simulink library "inp"  (R2021b)
settings: Solver=VariableStepAuto  StartTime=0.0  StopTime=10.0  RelTol=1e-3
undefined symbols (not defined in the file): C_TASK_5MS_S, FALSE, KINP_AcoreReadyToSlp_flg_ovrdflg, KINP_AcoreReadyToSlp_flg_ovrdval, KINP_AllowMovThd_OTA_enum_ovrdflg, KINP_AllowMovThd_OTA_enum_ovrdval, KINP_APSAngleTarget_Deg_ovrdflg, KINP_APSAngleTarget_Deg_ovrdval, KINP_APSDecReq_mps2_ovrdflg, KINP_APSDecReq_mps2_ovrdval, KINP_APSDecReqA_flg_ovrdflg, KINP_APSDecReqA_flg_ovrdval, KINP_APSDFLL_cm_ovrdflg, KINP_APSDFLL_cm_ovrdval, KINP_APSDFLR_cm_ovrdflg, KINP_APSDFLR_cm_ovrdval, KINP_APSDRLL_cm_ovrdflg, KINP_APSDRLL_cm_ovrdval, KINP_APSDRLR_cm_ovrdflg, KINP_APSDRLR_cm_ovrdval, KINP_APSExitCondition_enum_ovrdflg, KINP_APSExitCondition_enum_ovrdval, KINP_APSHWVer_enum_ovrdflg, KINP_APSHWVer_enum_ovrdval, KINP_APSProgressPCT_pct_ovrdflg, KINP_APSProgressPCT_pct_ovrdval, KINP_APSPwrReq_enum_ovrdflg, KINP_APSPwrReq_enum_ovrdval, KINP_APSReq_enum_ovrdflg, KINP_APSReq_enum_ovrdval, KINP_APSRQDisplay_enum_ovrdflg, KINP_APSRQDisplay_enum_ovrdval, KINP_APSRqEPASCtrl_flg_ovrdflg, KINP_APSRqEPASCtrl_flg_ovrdval, KINP_APSShiftPosnReq_enum_ovrdval, KINP_APSShiftPosnReq_enum_ovrflg, KINP_APSSpeedCMD_kph_ovrdval, KINP_APSSpeedCMD_kph_ovrflg, KINP_APSStaSystem_enum_ovrdflg, KINP_APSStaSystem_enum_ovrdval, KINP_APSSWVer_enum_ovrdflg, KINP_APSSWVer_enum_ovrdval, KINP_APSVMCReqA_flg_ovrdval, KINP_APSVMCReqA_flg_ovrflg, KINP_APSVRqEPASCtrl_flg_ovrdflg, KINP_APSVRqEPASCtrl_flg_ovrdval, KINP_AuxBattVolmV_mV_ovrdflg, KINP_AuxBattVolmV_mV_ovrdval, KINP_CAASSta_enum_ovrdflg, KINP_CAASSta_enum_ovrdval, KINP_CAASVMCReqA_flg_ovrdval, KINP_CAASVMCReqA_flg_ovrflg, KINP_CAN1BusOff_flg_ovrdflg, KINP_CAN1BusOff_flg_ovrdval, KINP_CAN2BusOff_flg_ovrdflg, KINP_CAN2BusOff_flg_ovrdval, KINP_CAN3BusOff_flg_ovrdflg, KINP_CAN3BusOff_flg_ovrdval, KINP_CAN4BusOff_flg_ovrdflg, KINP_CAN4BusOff_flg_ovrdval ... (+152)
libraries: FVT_lib x1035, hcu_lib x1
(part 28 of 33)

== system inp/INP/CAN4/SignalCheck/ZONE_FR_VCU ==
  BHAL_outputs : Inport
  inp_CanValid_bus : Inport  Port=2
  AGSErr : FVT_lib/inp/can_signal_template  SystemSampleTime=-1  VariantActivationTime=update diagram  Latency=0  AutoFrameSizeCalculation=off
      link override defval: Value=KINP_AGSErr_enum_defval
      link override ovrdflg: Value=KINP_AGSErr_enum_ovrdflg
      link override ovrdval: Value=KINP_AGSErr_enum_ovrdval
  BatInTemp : FVT_lib/inp/can_signal_template  SystemSampleTime=-1  VariantActivationTime=update diagram  Latency=0  AutoFrameSizeCalculation=off
      link override defval: Value=KINP_BatInTemp_C_defval
      link override ovrdflg: Value=KINP_BatInTemp_C_ovrdflg
      link override ovrdval: Value=KINP_BatInTemp_C_ovrdval
  BatInTempErr : FVT_lib/inp/can_signal_template  SystemSampleTime=-1  VariantActivationTime=update diagram  Latency=0  AutoFrameSizeCalculation=off
      link override defval: Value=KINP_BatInTempErr_enum_defval
      link override ovrdflg: Value=KINP_BatInTempErr_enum_ovrdflg
      link override ovrdval: Value=KINP_BatInTempErr_enum_ovrdval
  BatOutTemp : FVT_lib/inp/can_signal_template  SystemSampleTime=-1  VariantActivationTime=update diagram  Latency=0  AutoFrameSizeCalculation=off
      link override defval: Value=KINP_BatOutTemp_C_defval
      link override ovrdflg: Value=KINP_BatOutTemp_C_ovrdflg
      link override ovrdval: Value=KINP_BatOutTemp_C_ovrdval
  COMPErr : FVT_lib/inp/can_signal_template  SystemSampleTime=-1  VariantActivationTime=update diagram  Latency=0  AutoFrameSizeCalculation=off
      link override defval: Value=KINP_COMPErr_enum_defval
      link override ovrdflg: Value=KINP_COMPErr_enum_ovrdflg
      link override ovrdval: Value=KINP_COMPErr_enum_ovrdval
  EACProtectEnable : FVT_lib/inp/can_signal_template  SystemSampleTime=-1  VariantActivationTime=update diagram  Latency=0  AutoFrameSizeCalculation=off
      link override defval: Value=KINP_EACProtectEnable_enum_defval
      link override ovrdflg: Value=KINP_EACProtectEnable_enum_ovrdflg
      link override ovrdval: Value=KINP_EACProtectEnable_enum_ovrdval
  EWP3Err : FVT_lib/inp/can_signal_template  SystemSampleTime=-1  VariantActivationTime=update diagram  Latency=0  AutoFrameSizeCalculation=off
      link override defval: Value=KINP_EWP3Err_enum_defval
      link override ovrdflg: Value=KINP_EWP3Err_enum_ovrdflg
      link override ovrdval: Value=KINP_EWP3Err_enum_ovrdval
  EXV1Err : FVT_lib/inp/can_signal_template  SystemSampleTime=-1  VariantActivationTime=update diagram  Latency=0  AutoFrameSizeCalculation=off
      link override defval: Value=KINP_EXV1Err_enum_defval
      link override ovrdflg: Value=KINP_EXV1Err_enum_ovrdflg
      link override ovrdval: Value=KINP_EXV1Err_enum_ovrdval
  EXV2Err : FVT_lib/inp/can_signal_template  SystemSampleTime=-1  VariantActivationTime=update diagram  Latency=0  AutoFrameSizeCalculation=off
      link override defval: Value=KINP_EXV2Err_enum_defval
      link override ovrdflg: Value=KINP_EXV2Err_enum_ovrdflg
      link override ovrdval: Value=KINP_EXV2Err_enum_ovrdval
  FanErr : FVT_lib/inp/can_signal_template  SystemSampleTime=-1  VariantActivationTime=update diagram  Latency=0  AutoFrameSizeCalculation=off
      link override defval: Value=KINP_FanErr_enum_defval
      link override ovrdflg: Value=KINP_FanErr_enum_ovrdflg
      link override ovrdval: Value=KINP_FanErr_enum_ovrdval
  FrPMMLimpHomeActReq : FVT_lib/inp/can_signal_template  SystemSampleTime=-1  VariantActivationTime=update diagram  Latency=0  AutoFrameSizeCalculation=off
      link override defval: Value=KINP_FrPMMLimpHomeActReq_flg_defval
      link override ovrdflg: Value=KINP_FrPMMLimpHomeActReq_flg_ovrdflg
      link override ovrdval: Value=KINP_FrPMMLimpHomeActReq_flg_ovrdval
  MotorInTemp : FVT_lib/inp/can_signal_template  SystemSampleTime=-1  VariantActivationTime=update diagram  Latency=0  AutoFrameSizeCalculation=off
      link override defval: Value=KINP_MotorInTemp_C_defval
      link override ovrdflg: Value=KINP_MotorInTemp_C_ovrdflg
      link override ovrdval: Value=KINP_MotorInTemp_C_ovrdval
  MotorInTempErr : FVT_lib/inp/can_signal_template  SystemSampleTime=-1  VariantActivationTime=update diagram  Latency=0  AutoFrameSizeCalculation=off
      link override defval: Value=KINP_MotorInTempErr_enum_defval
      link override ovrdflg: Value=KINP_MotorInTempErr_enum_ovrdflg
      link override ovrdval: Value=KINP_MotorInTempErr_enum_ovrdval
  MotorOutTemp : FVT_lib/inp/can_signal_template  SystemSampleTime=-1  VariantActivationTime=update diagram  Latency=0  AutoFrameSizeCalculation=off
      link override defval: Value=KINP_MotorOutTemp_C_defval
      link override ovrdflg: Value=KINP_MotorOutTemp_C_ovrdflg
      link override ovrdval: Value=KINP_MotorOutTemp_C_ovrdval
  MotorOutTempErr : FVT_lib/inp/can_signal_template  SystemSampleTime=-1  VariantActivationTime=update diagram  Latency=0  AutoFrameSizeCalculation=off
      link override defval: Value=KINP_MotorOutTempErr_enum_defval
      link override ovrdflg: Value=KINP_MotorOutTempErr_enum_ovrdflg
      link override ovrdval: Value=KINP_MotorOutTempErr_enum_ovrdval
  PTHighP : FVT_lib/inp/can_signal_template  SystemSampleTime=-1  VariantActivationTime=update diagram  Latency=0  AutoFrameSizeCalculation=off
      link override defval: Value=KINP_PTHighP_KPa_defval
      link override ovrdflg: Value=KINP_PTHighP_KPa_ovrdflg
      link override ovrdval: Value=KINP_PTHighP_KPa_ovrdval
  PTHighPErr : FVT_lib/inp/can_signal_template  SystemSampleTime=-1  VariantActivationTime=update diagram  Latency=0  AutoFrameSizeCalculation=off
      link override defval: Value=KINP_PTHighPErr_enum_defval
      link override ovrdflg: Value=KINP_PTHighPErr_enum_ovrdflg
      link override ovrdval: Value=KINP_PTHighPErr_enum_ovrdval
  PTHighTact : FVT_lib/inp/can_signal_template  SystemSampleTime=-1  VariantActivationTime=update diagram  Latency=0  AutoFrameSizeCalculation=off
      link override defval: Value=KINP_PTHighTact_C_defval
      link override ovrdflg: Value=KINP_PTHighTact_C_ovrdflg
      link override ovrdval: Value=KINP_PTHighTact_C_ovrdval
  PTHighTactErr : FVT_lib/inp/can_signal_template  SystemSampleTime=-1  VariantActivationTime=update diagram  Latency=0  AutoFrameSizeCalculation=off
      link override defval: Value=KINP_PTHighTactErr_enum_defval
      link override ovrdflg: Value=KINP_PTHighTactErr_enum_ovrdflg
      link override ovrdval: Value=KINP_PTHighTactErr_enum_ovrdval
  PTLowP1 : FVT_lib/inp/can_signal_template  SystemSampleTime=-1  VariantActivationTime=update diagram  Latency=0  AutoFrameSizeCalculation=off
      link override defval: Value=KINP_PTLowP1_KPa_defval
      link override ovrdflg: Value=KINP_PTLowP1_KPa_ovrdflg
      link override ovrdval: Value=KINP_PTLowP1_KPa_ovrdval
  PTLowP1Err : FVT_lib/inp/can_signal_template  SystemSampleTime=-1  VariantActivationTime=update diagram  Latency=0  AutoFrameSizeCalculation=off
      link override defval: Value=KINP_PTLowP1Err_enum_defval
      link override ovrdflg: Value=KINP_PTLowP1Err_enum_ovrdflg
      link override ovrdval: Value=KINP_PTLowP1Err_enum_ovrdval
  PTLowP2 : FVT_lib/inp/can_signal_template  SystemSampleTime=-1  VariantActivationTime=update diagram  Latency=0  AutoFrameSizeCalculation=off
      link override defval: Value=KINP_PTLowP2_KPa_defval
      link override ovrdflg: Value=KINP_PTLowP2_KPa_ovrdflg
      link override ovrdval: Value=KINP_PTLowP2_KPa_ovrdval
  PTLowP2Err : FVT_lib/inp/can_signal_template  SystemSampleTime=-1  VariantActivationTime=update diagram  Latency=0  AutoFrameSizeCalculation=off
      link override defval: Value=KINP_PTLowP2Err_enum_defval
      link override ovrdflg: Value=KINP_PTLowP2Err_enum_ovrdflg
      link override ovrdval: Value=KINP_PTLowP2Err_enum_ovrdval
  PTLowT1 : FVT_lib/inp/can_signal_template  SystemSampleTime=-1  VariantActivationTime=update diagram  Latency=0  AutoFrameSizeCalculation=off
      link override defval: Value=KINP_PTLowT1_C_defval
      link override ovrdflg: Value=KINP_PTLowT1_C_ovrdflg
      link override ovrdval: Value=KINP_PTLowT1_C_ovrdval
  PTLowT1Err : FVT_lib/inp/can_signal_template  SystemSampleTime=-1  VariantActivationTime=update diagram  Latency=0  AutoFrameSizeCalculation=off
      link override defval: Value=KINP_PTLowT1Err_enum_defval
      link override ovrdflg: Value=KINP_PTLowT1Err_enum_ovrdflg
      link override ovrdval: Value=KINP_PTLowT1Err_enum_ovrdval
  PTLowT2 : FVT_lib/inp/can_signal_template  SystemSampleTime=-1  VariantActivationTime=update diagram  Latency=0  AutoFrameSizeCalculation=off
      link override defval: Value=KINP_PTLowT2_C_defval
      link override ovrdflg: Value=KINP_PTLowT2_C_ovrdflg
      link override ovrdval: Value=KINP_PTLowT2_C_ovrdval
  PTLowT2Err : FVT_lib/inp/can_signal_template  SystemSampleTime=-1  VariantActivationTime=update diagram  Latency=0  AutoFrameSizeCalculation=off
      link override defval: Value=KINP_PTLowT2Err_enum_defval
      link override ovrdflg: Value=KINP_PTLowT2Err_enum_ovrdflg
      link override ovrdval: Value=KINP_PTLowT2Err_enum_ovrdval
  SOTXVErr : FVT_lib/inp/can_signal_template  SystemSampleTime=-1  VariantActivationTime=update diagram  Latency=0  AutoFrameSizeCalculation=off
      link override defval: Value=KINP_SOTXVErr_enum_defval
      link override ovrdflg: Value=KINP_SOTXVErr_enum_ovrdflg
      link override ovrdval: Value=KINP_SOTXVErr_enum_ovrdval
  SOV1Err : FVT_lib/inp/can_signal_template  SystemSampleTime=-1  VariantActivationTime=update diagram  Latency=0  AutoFrameSizeCalculation=off
      link override defval: Value=KINP_SOV1Err_enum_defval
      link override ovrdflg: Value=KINP_SOV1Err_enum_ovrdflg
      link override ovrdval: Value=KINP_SOV1Err_enum_ovrdval
  SOV2Err : FVT_lib/inp/can_signal_template  SystemSampleTime=-1  VariantActivationTime=update diagram  Latency=0  AutoFrameSizeCalculation=off
      link override defval: Value=KINP_SOV2Err_enum_defval
      link override ovrdflg: Value=KINP_SOV2Err_enum_ovrdflg
      link override ovrdval: Value=KINP_SOV2Err_enum_ovrdval
  SOV3Err : FVT_lib/inp/can_signal_template  SystemSampleTime=-1  VariantActivationTime=update diagram  Latency=0  AutoFrameSizeCalculation=off
      link override defval: Value=KINP_SOV3Err_enum_defval
      link override ovrdflg: Value=KINP_SOV3Err_enum_ovrdflg
      link override ovrdval: Value=KINP_SOV3Err_enum_ovrdval
  Tamb : FVT_lib/inp/can_signal_template  SystemSampleTime=-1  VariantActivationTime=update diagram  Latency=0  AutoFrameSizeCalculation=off
      link override defval: Value=KINP_Tamb_C_defval
      link override ovrdflg: Value=KINP_Tamb_C_ovrdflg
      link override ovrdval: Value=KINP_Tamb_C_ovrdval
  TambErr : FVT_lib/inp/can_signal_template  SystemSampleTime=-1  VariantActivationTime=update diagram  Latency=0  AutoFrameSizeCalculation=off
      link override defval: Value=KINP_TambErr_enum_defval
      link override ovrdflg: Value=KINP_TambErr_enum_ovrdflg
      link override ovrdval: Value=KINP_TambErr_enum_ovrdval
  Terminator_{1..33} (33 alike) : Terminator
  True_VHAL_AGSErr_enum : Constant  Value=TRUE  OutDataTypeStr=boolean
  True_VHAL_BatInTempErr_enum : Constant  Value=TRUE  OutDataTypeStr=boolean
  True_VHAL_BatInTemp_C : Constant  Value=TRUE  OutDataTypeStr=boolean
  True_VHAL_BatOutTemp_C : Constant  Value=TRUE  OutDataTypeStr=boolean
  True_VHAL_COMPErr_enum : Constant  Value=TRUE  OutDataTypeStr=boolean
  True_VHAL_EACProtectEnable_enum : Constant  Value=TRUE  OutDataTypeStr=boolean
  True_VHAL_EWP3Err_enum : Constant  Value=TRUE  OutDataTypeStr=boolean
  True_VHAL_EXV1Err_enum : Constant  Value=TRUE  OutDataTypeStr=boolean
  True_VHAL_EXV2Err_enum : Constant  Value=TRUE  OutDataTypeStr=boolean
  True_VHAL_FanErr_enum : Constant  Value=TRUE  OutDataTypeStr=boolean
  True_VHAL_FrPMMLimpHomeActReq_flg : Constant  Value=TRUE  OutDataTypeStr=boolean
  True_VHAL_MotorInTempErr_enum : Constant  Value=TRUE  OutDataTypeStr=boolean
  True_VHAL_MotorInTemp_C : Constant  Value=TRUE  OutDataTypeStr=boolean
  True_VHAL_MotorOutTempErr_enum : Constant  Value=TRUE  OutDataTypeStr=boolean
  True_VHAL_MotorOutTemp_C : Constant  Value=TRUE  OutDataTypeStr=boolean
  True_VHAL_PTHighPErr_enum : Constant  Value=TRUE  OutDataTypeStr=boolean
  True_VHAL_PTHighP_KPa : Constant  Value=TRUE  OutDataTypeStr=boolean
  True_VHAL_PTHighTactErr_enum : Constant  Value=TRUE  OutDataTypeStr=boolean
  True_VHAL_PTHighTact_C : Constant  Value=TRUE  OutDataTypeStr=boolean
  True_VHAL_PTLowP1Err_enum : Constant  Value=TRUE  OutDataTypeStr=boolean
  True_VHAL_PTLowP1_KPa : Constant  Value=TRUE  OutDataTypeStr=boolean
  True_VHAL_PTLowP2Err_enum : Constant  Value=TRUE  OutDataTypeStr=boolean
  True_VHAL_PTLowP2_KPa : Constant  Value=TRUE  OutDataTypeStr=boolean
  True_VHAL_PTLowT1Err_enum : Constant  Value=TRUE  OutDataTypeStr=boolean
  True_VHAL_PTLowT1_C : Constant  Value=TRUE  OutDataTypeStr=boolean
  True_VHAL_PTLowT2Err_enum : Constant  Value=TRUE  OutDataTypeStr=boolean
  True_VHAL_PTLowT2_C : Constant  Value=TRUE  OutDataTypeStr=boolean
  True_VHAL_SOTXVErr_enum : Constant  Value=TRUE  OutDataTypeStr=boolean
  True_VHAL_SOV1Err_enum : Constant  Value=TRUE  OutDataTypeStr=boolean
  True_VHAL_SOV2Err_enum : Constant  Value=TRUE  OutDataTypeStr=boolean
  True_VHAL_SOV3Err_enum : Constant  Value=TRUE  OutDataTypeStr=boolean
  True_VHAL_TambErr_enum : Constant  Value=TRUE  OutDataTypeStr=boolean
  True_VHAL_Tamb_C : Constant  Value=TRUE  OutDataTypeStr=boolean
  slr1_{1..33} (33 alike) : BusSelector  OutputSignals=VINP_CANMsgValidZONEFRVCU_flg
  slr_VHAL_AGSErr_enum : BusSelector  OutputSignals=VHAL_AGSErr_enum
  slr_VHAL_BatInTempErr_enum : BusSelector  OutputSignals=VHAL_BatInTempErr_enum
  slr_VHAL_BatInTemp_C : BusSelector  OutputSignals=VHAL_BatInTemp_C
  slr_VHAL_BatOutTemp_C : BusSelector  OutputSignals=VHAL_BatOutTemp_C
  slr_VHAL_COMPErr_enum : BusSelector  OutputSignals=VHAL_COMPErr_enum
  slr_VHAL_EACProtectEnable_enum : BusSelector  OutputSignals=VHAL_EACProtectEnable_enum
  slr_VHAL_EWP3Err_enum : BusSelector  OutputSignals=VHAL_EWP3Err_enum
  slr_VHAL_EXV1Err_enum : BusSelector  OutputSignals=VHAL_EXV1Err_enum
  slr_VHAL_EXV2Err_enum : BusSelector  OutputSignals=VHAL_EXV2Err_enum
  slr_VHAL_FanErr_enum : BusSelector  OutputSignals=VHAL_FanErr_enum
  slr_VHAL_FrPMMLimpHomeActReq_flg : BusSelector  OutputSignals=VHAL_FrPMMLimpHomeActReq_flg
  slr_VHAL_MotorInTempErr_enum : BusSelector  OutputSignals=VHAL_MotorInTempErr_enum
  slr_VHAL_MotorInTemp_C : BusSelector  OutputSignals=VHAL_MotorInTemp_C
  slr_VHAL_MotorOutTempErr_enum : BusSelector  OutputSignals=VHAL_MotorOutTempErr_enum
  slr_VHAL_MotorOutTemp_C : BusSelector  OutputSignals=VHAL_MotorOutTemp_C
  slr_VHAL_PTHighPErr_enum : BusSelector  OutputSignals=VHAL_PTHighPErr_enum
  slr_VHAL_PTHighP_KPa : BusSelector  OutputSignals=VHAL_PTHighP_KPa
  slr_VHAL_PTHighTactErr_enum : BusSelector  OutputSignals=VHAL_PTHighTactErr_enum
  slr_VHAL_PTHighTact_C : BusSelector  OutputSignals=VHAL_PTHighTact_C
  slr_VHAL_PTLowP1Err_enum : BusSelector  OutputSignals=VHAL_PTLowP1Err_enum
  slr_VHAL_PTLowP1_KPa : BusSelector  OutputSignals=VHAL_PTLowP1_KPa
  slr_VHAL_PTLowP2Err_enum : BusSelector  OutputSignals=VHAL_PTLowP2Err_enum
  slr_VHAL_PTLowP2_KPa : BusSelector  OutputSignals=VHAL_PTLowP2_KPa
  slr_VHAL_PTLowT1Err_enum : BusSelector  OutputSignals=VHAL_PTLowT1Err_enum
  slr_VHAL_PTLowT1_C : BusSelector  OutputSignals=VHAL_PTLowT1_C
  slr_VHAL_PTLowT2Err_enum : BusSelector  OutputSignals=VHAL_PTLowT2Err_enum
  slr_VHAL_PTLowT2_C : BusSelector  OutputSignals=VHAL_PTLowT2_C
  slr_VHAL_SOTXVErr_enum : BusSelector  OutputSignals=VHAL_SOTXVErr_enum
  slr_VHAL_SOV1Err_enum : BusSelector  OutputSignals=VHAL_SOV1Err_enum
  slr_VHAL_SOV2Err_enum : BusSelector  OutputSignals=VHAL_SOV2Err_enum
  slr_VHAL_SOV3Err_enum : BusSelector  OutputSignals=VHAL_SOV3Err_enum
  slr_VHAL_TambErr_enum : BusSelector  OutputSignals=VHAL_TambErr_enum
  slr_VHAL_Tamb_C : BusSelector  OutputSignals=VHAL_Tamb_C
  VINP_AGSErr_enum : Outport
  VINP_BatInTemp_C : Outport  Port=2
  VINP_BatInTempErr_enum : Outport  Port=3
  VINP_BatOutTemp_C : Outport  Port=4
  VINP_COMPErr_enum : Outport  Port=5
  VINP_EACProtectEnable_enum : Outport  Port=6
  VINP_EWP3Err_enum : Outport  Port=7
  VINP_EXV1Err_enum : Outport  Port=8
  VINP_EXV2Err_enum : Outport  Port=9
  VINP_FanErr_enum : Outport  Port=10
  VINP_FrPMMLimpHomeActReq_flg : Outport  Port=11
  VINP_MotorInTemp_C : Outport  Port=12
  VINP_MotorInTempErr_enum : Outport  Port=13
  VINP_MotorOutTemp_C : Outport  Port=14
  VINP_MotorOutTempErr_enum : Outport  Port=15
  VINP_PTHighP_KPa : Outport  Port=16
  VINP_PTHighPErr_enum : Outport  Port=17
  VINP_PTHighTact_C : Outport  Port=18
  VINP_PTHighTactErr_enum : Outport  Port=19
  VINP_PTLowP1_KPa : Outport  Port=20
  VINP_PTLowP1Err_enum : Outport  Port=21
  VINP_PTLowP2_KPa : Outport  Port=22
  VINP_PTLowP2Err_enum : Outport  Port=23
  VINP_PTLowT1_C : Outport  Port=24
  VINP_PTLowT1Err_enum : Outport  Port=25
  VINP_PTLowT2_C : Outport  Port=26
  VINP_PTLowT2Err_enum : Outport  Port=27
  VINP_SOTXVErr_enum : Outport  Port=28
  VINP_SOV1Err_enum : Outport  Port=29
  VINP_SOV2Err_enum : Outport  Port=30
  VINP_SOV3Err_enum : Outport  Port=31
  VINP_Tamb_C : Outport  Port=32
  VINP_TambErr_enum : Outport  Port=33
  wires:
  BHAL_outputs/1 -> [BHAL_outputs]
  inp_CanValid_bus/1 -> [inp_CanValid_bus]
  [BHAL_outputs] -> slr_VHAL_AGSErr_enum/1
  slr_VHAL_AGSErr_enum/1 -> AGSErr/1  "<VHAL_AGSErr_enum>"
  True_VHAL_AGSErr_enum/1 -> AGSErr/2
  [inp_CanValid_bus] -> slr1_1/1
  slr1_1/1 -> AGSErr/3  "<VINP_CANMsgValidZONEFRVCU_flg>"
  AGSErr/1 -> VINP_AGSErr_enum/1  "VINP_AGSErr_enum"
  AGSErr/2 -> Terminator_1/1
  [BHAL_outputs] -> slr_VHAL_BatInTemp_C/1
  slr_VHAL_BatInTemp_C/1 -> BatInTemp/1  "<VHAL_BatInTemp_C>"
  True_VHAL_BatInTemp_C/1 -> BatInTemp/2
  [inp_CanValid_bus] -> slr1_2/1
  slr1_2/1 -> BatInTemp/3  "<VINP_CANMsgValidZONEFRVCU_flg>"
  BatInTemp/1 -> VINP_BatInTemp_C/1  "VINP_BatInTemp_C"
  BatInTemp/2 -> Terminator_2/1
  [BHAL_outputs] -> slr_VHAL_BatInTempErr_enum/1
  slr_VHAL_BatInTempErr_enum/1 -> BatInTempErr/1  "<VHAL_BatInTempErr_enum>"
  True_VHAL_BatInTempErr_enum/1 -> BatInTempErr/2
  [inp_CanValid_bus] -> slr1_3/1
  slr1_3/1 -> BatInTempErr/3  "<VINP_CANMsgValidZONEFRVCU_flg>"
  BatInTempErr/1 -> VINP_BatInTempErr_enum/1  "VINP_BatInTempErr_enum"
  BatInTempErr/2 -> Terminator_3/1
  [BHAL_outputs] -> slr_VHAL_BatOutTemp_C/1
  slr_VHAL_BatOutTemp_C/1 -> BatOutTemp/1  "<VHAL_BatOutTemp_C>"
  True_VHAL_BatOutTemp_C/1 -> BatOutTemp/2
  [inp_CanValid_bus] -> slr1_4/1
  slr1_4/1 -> BatOutTemp/3  "<VINP_CANMsgValidZONEFRVCU_flg>"
  BatOutTemp/1 -> VINP_BatOutTemp_C/1  "VINP_BatOutTemp_C"
  BatOutTemp/2 -> Terminator_4/1
  [BHAL_outputs] -> slr_VHAL_COMPErr_enum/1
  slr_VHAL_COMPErr_enum/1 -> COMPErr/1  "<VHAL_COMPErr_enum>"
  True_VHAL_COMPErr_enum/1 -> COMPErr/2
  [inp_CanValid_bus] -> slr1_5/1
  slr1_5/1 -> COMPErr/3  "<VINP_CANMsgValidZONEFRVCU_flg>"
  COMPErr/1 -> VINP_COMPErr_enum/1  "VINP_COMPErr_enum"
  COMPErr/2 -> Terminator_5/1
  [BHAL_outputs] -> slr_VHAL_EACProtectEnable_enum/1
  slr_VHAL_EACProtectEnable_enum/1 -> EACProtectEnable/1  "<VHAL_EACProtectEnable_enum>"
  True_VHAL_EACProtectEnable_enum/1 -> EACProtectEnable/2
  [inp_CanValid_bus] -> slr1_6/1
  slr1_6/1 -> EACProtectEnable/3  "<VINP_CANMsgValidZONEFRVCU_flg>"
  EACProtectEnable/1 -> VINP_EACProtectEnable_enum/1  "VINP_EACProtectEnable_enum"
  EACProtectEnable/2 -> Terminator_6/1
  [BHAL_outputs] -> slr_VHAL_EWP3Err_enum/1
  slr_VHAL_EWP3Err_enum/1 -> EWP3Err/1  "<VHAL_EWP3Err_enum>"
  True_VHAL_EWP3Err_enum/1 -> EWP3Err/2
  [inp_CanValid_bus] -> slr1_7/1
  slr1_7/1 -> EWP3Err/3  "<VINP_CANMsgValidZONEFRVCU_flg>"
  EWP3Err/1 -> VINP_EWP3Err_enum/1  "VINP_EWP3Err_enum"
  EWP3Err/2 -> Terminator_7/1
  [BHAL_outputs] -> slr_VHAL_EXV1Err_enum/1
  slr_VHAL_EXV1Err_enum/1 -> EXV1Err/1  "<VHAL_EXV1Err_enum>"
  True_VHAL_EXV1Err_enum/1 -> EXV1Err/2
  [inp_CanValid_bus] -> slr1_8/1
  slr1_8/1 -> EXV1Err/3  "<VINP_CANMsgValidZONEFRVCU_flg>"
  EXV1Err/1 -> VINP_EXV1Err_enum/1  "VINP_EXV1Err_enum"
  EXV1Err/2 -> Terminator_8/1
  [BHAL_outputs] -> slr_VHAL_EXV2Err_enum/1
  slr_VHAL_EXV2Err_enum/1 -> EXV2Err/1  "<VHAL_EXV2Err_enum>"
  True_VHAL_EXV2Err_enum/1 -> EXV2Err/2
  [inp_CanValid_bus] -> slr1_9/1
  slr1_9/1 -> EXV2Err/3  "<VINP_CANMsgValidZONEFRVCU_flg>"
  EXV2Err/1 -> VINP_EXV2Err_enum/1  "VINP_EXV2Err_enum"
  EXV2Err/2 -> Terminator_9/1
  [BHAL_outputs] -> slr_VHAL_FanErr_enum/1
  slr_VHAL_FanErr_enum/1 -> FanErr/1  "<VHAL_FanErr_enum>"
  True_VHAL_FanErr_enum/1 -> FanErr/2
  [inp_CanValid_bus] -> slr1_10/1
  slr1_10/1 -> FanErr/3  "<VINP_CANMsgValidZONEFRVCU_flg>"
  FanErr/1 -> VINP_FanErr_enum/1  "VINP_FanErr_enum"
  FanErr/2 -> Terminator_10/1
  [BHAL_outputs] -> slr_VHAL_FrPMMLimpHomeActReq_flg/1
  slr_VHAL_FrPMMLimpHomeActReq_flg/1 -> FrPMMLimpHomeActReq/1  "<VHAL_FrPMMLimpHomeActReq_flg>"
  True_VHAL_FrPMMLimpHomeActReq_flg/1 -> FrPMMLimpHomeActReq/2
  [inp_CanValid_bus] -> slr1_11/1
  slr1_11/1 -> FrPMMLimpHomeActReq/3  "<VINP_CANMsgValidZONEFRVCU_flg>"
  FrPMMLimpHomeActReq/1 -> VINP_FrPMMLimpHomeActReq_flg/1  "VINP_FrPMMLimpHomeActReq_flg"
  FrPMMLimpHomeActReq/2 -> Terminator_11/1
  [BHAL_outputs] -> slr_VHAL_MotorInTemp_C/1
  slr_VHAL_MotorInTemp_C/1 -> MotorInTemp/1  "<VHAL_MotorInTemp_C>"
  True_VHAL_MotorInTemp_C/1 -> MotorInTemp/2
  [inp_CanValid_bus] -> slr1_12/1
  slr1_12/1 -> MotorInTemp/3  "<VINP_CANMsgValidZONEFRVCU_flg>"
  MotorInTemp/1 -> VINP_MotorInTemp_C/1  "VINP_MotorInTemp_C"
  MotorInTemp/2 -> Terminator_12/1
  [BHAL_outputs] -> slr_VHAL_MotorInTempErr_enum/1
  slr_VHAL_MotorInTempErr_enum/1 -> MotorInTempErr/1  "<VHAL_MotorInTempErr_enum>"
  True_VHAL_MotorInTempErr_enum/1 -> MotorInTempErr/2
  [inp_CanValid_bus] -> slr1_13/1
  slr1_13/1 -> MotorInTempErr/3  "<VINP_CANMsgValidZONEFRVCU_flg>"
  MotorInTempErr/1 -> VINP_MotorInTempErr_enum/1  "VINP_MotorInTempErr_enum"
  MotorInTempErr/2 -> Terminator_13/1
  [BHAL_outputs] -> slr_VHAL_MotorOutTemp_C/1
  slr_VHAL_MotorOutTemp_C/1 -> MotorOutTemp/1  "<VHAL_MotorOutTemp_C>"
  True_VHAL_MotorOutTemp_C/1 -> MotorOutTemp/2
  [inp_CanValid_bus] -> slr1_14/1
  slr1_14/1 -> MotorOutTemp/3  "<VINP_CANMsgValidZONEFRVCU_flg>"
  MotorOutTemp/1 -> VINP_MotorOutTemp_C/1  "VINP_MotorOutTemp_C"
  MotorOutTemp/2 -> Terminator_14/1
  [BHAL_outputs] -> slr_VHAL_MotorOutTempErr_enum/1
  slr_VHAL_MotorOutTempErr_enum/1 -> MotorOutTempErr/1  "<VHAL_MotorOutTempErr_enum>"
  True_VHAL_MotorOutTempErr_enum/1 -> MotorOutTempErr/2
  [inp_CanValid_bus] -> slr1_15/1
  slr1_15/1 -> MotorOutTempErr/3  "<VINP_CANMsgValidZONEFRVCU_flg>"
  MotorOutTempErr/1 -> VINP_MotorOutTempErr_enum/1  "VINP_MotorOutTempErr_enum"
  MotorOutTempErr/2 -> Terminator_15/1
  [BHAL_outputs] -> slr_VHAL_PTHighP_KPa/1
  slr_VHAL_PTHighP_KPa/1 -> PTHighP/1  "<VHAL_PTHighP_KPa>"
  True_VHAL_PTHighP_KPa/1 -> PTHighP/2
  [inp_CanValid_bus] -> slr1_16/1
  slr1_16/1 -> PTHighP/3  "<VINP_CANMsgValidZONEFRVCU_flg>"
  PTHighP/1 -> VINP_PTHighP_KPa/1  "VINP_PTHighP_KPa"
  PTHighP/2 -> Terminator_16/1
  [BHAL_outputs] -> slr_VHAL_PTHighPErr_enum/1
  slr_VHAL_PTHighPErr_enum/1 -> PTHighPErr/1  "<VHAL_PTHighPErr_enum>"
  True_VHAL_PTHighPErr_enum/1 -> PTHighPErr/2
  [inp_CanValid_bus] -> slr1_17/1
  slr1_17/1 -> PTHighPErr/3  "<VINP_CANMsgValidZONEFRVCU_flg>"
  PTHighPErr/1 -> VINP_PTHighPErr_enum/1  "VINP_PTHighPErr_enum"
  PTHighPErr/2 -> Terminator_17/1
  [BHAL_outputs] -> slr_VHAL_PTHighTact_C/1
  slr_VHAL_PTHighTact_C/1 -> PTHighTact/1  "<VHAL_PTHighTact_C>"
  True_VHAL_PTHighTact_C/1 -> PTHighTact/2
  [inp_CanValid_bus] -> slr1_18/1
  slr1_18/1 -> PTHighTact/3  "<VINP_CANMsgValidZONEFRVCU_flg>"
  PTHighTact/1 -> VINP_PTHighTact_C/1  "VINP_PTHighTact_C"
  PTHighTact/2 -> Terminator_18/1
  [BHAL_outputs] -> slr_VHAL_PTHighTactErr_enum/1
  slr_VHAL_PTHighTactErr_enum/1 -> PTHighTactErr/1  "<VHAL_PTHighTactErr_enum>"
  True_VHAL_PTHighTactErr_enum/1 -> PTHighTactErr/2
  [inp_CanValid_bus] -> slr1_19/1
  slr1_19/1 -> PTHighTactErr/3  "<VINP_CANMsgValidZONEFRVCU_flg>"
  PTHighTactErr/1 -> VINP_PTHighTactErr_enum/1  "VINP_PTHighTactErr_enum"
  PTHighTactErr/2 -> Terminator_19/1
  [BHAL_outputs] -> slr_VHAL_PTLowP1_KPa/1
  slr_VHAL_PTLowP1_KPa/1 -> PTLowP1/1  "<VHAL_PTLowP1_KPa>"
  True_VHAL_PTLowP1_KPa/1 -> PTLowP1/2
  [inp_CanValid_bus] -> slr1_20/1
  slr1_20/1 -> PTLowP1/3  "<VINP_CANMsgValidZONEFRVCU_flg>"
  PTLowP1/1 -> VINP_PTLowP1_KPa/1  "VINP_PTLowP1_KPa"
  PTLowP1/2 -> Terminator_20/1
  [BHAL_outputs] -> slr_VHAL_PTLowP1Err_enum/1
  slr_VHAL_PTLowP1Err_enum/1 -> PTLowP1Err/1  "<VHAL_PTLowP1Err_enum>"
  True_VHAL_PTLowP1Err_enum/1 -> PTLowP1Err/2
  [inp_CanValid_bus] -> slr1_21/1
  slr1_21/1 -> PTLowP1Err/3  "<VINP_CANMsgValidZONEFRVCU_flg>"
  PTLowP1Err/1 -> VINP_PTLowP1Err_enum/1  "VINP_PTLowP1Err_enum"
  PTLowP1Err/2 -> Terminator_21/1
  [BHAL_outputs] -> slr_VHAL_PTLowP2_KPa/1
  slr_VHAL_PTLowP2_KPa/1 -> PTLowP2/1  "<VHAL_PTLowP2_KPa>"
  True_VHAL_PTLowP2_KPa/1 -> PTLowP2/2
  [inp_CanValid_bus] -> slr1_22/1
  slr1_22/1 -> PTLowP2/3  "<VINP_CANMsgValidZONEFRVCU_flg>"
  PTLowP2/1 -> VINP_PTLowP2_KPa/1  "VINP_PTLowP2_KPa"
  PTLowP2/2 -> Terminator_22/1
  [BHAL_outputs] -> slr_VHAL_PTLowP2Err_enum/1
  slr_VHAL_PTLowP2Err_enum/1 -> PTLowP2Err/1  "<VHAL_PTLowP2Err_enum>"
  True_VHAL_PTLowP2Err_enum/1 -> PTLowP2Err/2
  [inp_CanValid_bus] -> slr1_23/1
  slr1_23/1 -> PTLowP2Err/3  "<VINP_CANMsgValidZONEFRVCU_flg>"
  PTLowP2Err/1 -> VINP_PTLowP2Err_enum/1  "VINP_PTLowP2Err_enum"
  PTLowP2Err/2 -> Terminator_23/1
  [BHAL_outputs] -> slr_VHAL_PTLowT1_C/1
  slr_VHAL_PTLowT1_C/1 -> PTLowT1/1  "<VHAL_PTLowT1_C>"
  True_VHAL_PTLowT1_C/1 -> PTLowT1/2
  [inp_CanValid_bus] -> slr1_24/1
  slr1_24/1 -> PTLowT1/3  "<VINP_CANMsgValidZONEFRVCU_flg>"
  PTLowT1/1 -> VINP_PTLowT1_C/1  "VINP_PTLowT1_C"
  PTLowT1/2 -> Terminator_24/1
  [BHAL_outputs] -> slr_VHAL_PTLowT1Err_enum/1
  slr_VHAL_PTLowT1Err_enum/1 -> PTLowT1Err/1  "<VHAL_PTLowT1Err_enum>"
  True_VHAL_PTLowT1Err_enum/1 -> PTLowT1Err/2
  [inp_CanValid_bus] -> slr1_25/1
  slr1_25/1 -> PTLowT1Err/3  "<VINP_CANMsgValidZONEFRVCU_flg>"
  PTLowT1Err/1 -> VINP_PTLowT1Err_enum/1  "VINP_PTLowT1Err_enum"
  PTLowT1Err/2 -> Terminator_25/1
  [BHAL_outputs] -> slr_VHAL_PTLowT2_C/1
  slr_VHAL_PTLowT2_C/1 -> PTLowT2/1  "<VHAL_PTLowT2_C>"
  True_VHAL_PTLowT2_C/1 -> PTLowT2/2
  [inp_CanValid_bus] -> slr1_26/1
  slr1_26/1 -> PTLowT2/3  "<VINP_CANMsgValidZONEFRVCU_flg>"
  PTLowT2/1 -> VINP_PTLowT2_C/1  "VINP_PTLowT2_C"
  PTLowT2/2 -> Terminator_26/1
  [BHAL_outputs] -> slr_VHAL_PTLowT2Err_enum/1
  slr_VHAL_PTLowT2Err_enum/1 -> PTLowT2Err/1  "<VHAL_PTLowT2Err_enum>"
  True_VHAL_PTLowT2Err_enum/1 -> PTLowT2Err/2
  [inp_CanValid_bus] -> slr1_27/1
  slr1_27/1 -> PTLowT2Err/3  "<VINP_CANMsgValidZONEFRVCU_flg>"
  PTLowT2Err/1 -> VINP_PTLowT2Err_enum/1  "VINP_PTLowT2Err_enum"
  PTLowT2Err/2 -> Terminator_27/1
  [BHAL_outputs] -> slr_VHAL_SOTXVErr_enum/1
  slr_VHAL_SOTXVErr_enum/1 -> SOTXVErr/1  "<VHAL_SOTXVErr_enum>"
  True_VHAL_SOTXVErr_enum/1 -> SOTXVErr/2
  [inp_CanValid_bus] -> slr1_28/1
  slr1_28/1 -> SOTXVErr/3  "<VINP_CANMsgValidZONEFRVCU_flg>"
  SOTXVErr/1 -> VINP_SOTXVErr_enum/1  "VINP_SOTXVErr_enum"
  SOTXVErr/2 -> Terminator_28/1
  [BHAL_outputs] -> slr_VHAL_SOV1Err_enum/1
  slr_VHAL_SOV1Err_enum/1 -> SOV1Err/1  "<VHAL_SOV1Err_enum>"
  True_VHAL_SOV1Err_enum/1 -> SOV1Err/2
  [inp_CanValid_bus] -> slr1_29/1
  slr1_29/1 -> SOV1Err/3  "<VINP_CANMsgValidZONEFRVCU_flg>"
  SOV1Err/1 -> VINP_SOV1Err_enum/1  "VINP_SOV1Err_enum"
  SOV1Err/2 -> Terminator_29/1
  [BHAL_outputs] -> slr_VHAL_SOV2Err_enum/1
  slr_VHAL_SOV2Err_enum/1 -> SOV2Err/1  "<VHAL_SOV2Err_enum>"
  True_VHAL_SOV2Err_enum/1 -> SOV2Err/2
  [inp_CanValid_bus] -> slr1_30/1
  slr1_30/1 -> SOV2Err/3  "<VINP_CANMsgValidZONEFRVCU_flg>"
  SOV2Err/1 -> VINP_SOV2Err_enum/1  "VINP_SOV2Err_enum"
  SOV2Err/2 -> Terminator_30/1
  [BHAL_outputs] -> slr_VHAL_SOV3Err_enum/1
  slr_VHAL_SOV3Err_enum/1 -> SOV3Err/1  "<VHAL_SOV3Err_enum>"
  True_VHAL_SOV3Err_enum/1 -> SOV3Err/2
  [inp_CanValid_bus] -> slr1_31/1
  slr1_31/1 -> SOV3Err/3  "<VINP_CANMsgValidZONEFRVCU_flg>"
  SOV3Err/1 -> VINP_SOV3Err_enum/1  "VINP_SOV3Err_enum"
  SOV3Err/2 -> Terminator_31/1
  [BHAL_outputs] -> slr_VHAL_Tamb_C/1
  slr_VHAL_Tamb_C/1 -> Tamb/1  "<VHAL_Tamb_C>"
  True_VHAL_Tamb_C/1 -> Tamb/2
  [inp_CanValid_bus] -> slr1_32/1
  slr1_32/1 -> Tamb/3  "<VINP_CANMsgValidZONEFRVCU_flg>"
  Tamb/1 -> VINP_Tamb_C/1  "VINP_Tamb_C"
  Tamb/2 -> Terminator_32/1
  [BHAL_outputs] -> slr_VHAL_TambErr_enum/1
  slr_VHAL_TambErr_enum/1 -> TambErr/1  "<VHAL_TambErr_enum>"
  True_VHAL_TambErr_enum/1 -> TambErr/2
  [inp_CanValid_bus] -> slr1_33/1
  slr1_33/1 -> TambErr/3  "<VINP_CANMsgValidZONEFRVCU_flg>"
  TambErr/1 -> VINP_TambErr_enum/1  "VINP_TambErr_enum"
  TambErr/2 -> Terminator_33/1

== system inp/INP/CAN4/SignalCheck/zGW_APTC1 ==
  BHAL_outputs : Inport
  inp_CanValid_bus : Inport  Port=2
  FrntPTCLeActHeatPwr : FVT_lib/inp/can_signal_template  SystemSampleTime=-1  VariantActivationTime=update diagram  Latency=0  AutoFrameSizeCalculation=off
      link override defval: Value=KINP_FrntPTCLeActHeatPwr_W_defval
      link override ovrdflg: Value=KINP_FrntPTCLeActHeatPwr_W_ovrdflg
      link override ovrdval: Value=KINP_FrntPTCLeActHeatPwr_W_ovrdval
  FrntPTCRearLeActHeatPwr : FVT_lib/inp/can_signal_template  SystemSampleTime=-1  VariantActivationTime=update diagram  Latency=0  AutoFrameSizeCalculation=off
      link override defval: Value=KINP_FrntPTCRearLeActHeatPwr_W_defval
      link override ovrdflg: Value=KINP_FrntPTCRearLeActHeatPwr_W_ovrdflg
      link override ovrdval: Value=KINP_FrntPTCRearLeActHeatPwr_W_ovrdval
  FrntPTCRearRiActHeatPwr : FVT_lib/inp/can_signal_template  SystemSampleTime=-1  VariantActivationTime=update diagram  Latency=0  AutoFrameSizeCalculation=off
      link override defval: Value=KINP_FrntPTCRearRiActHeatPwr_W_defval
      link override ovrdflg: Value=KINP_FrntPTCRearRiActHeatPwr_W_ovrdflg
      link override ovrdval: Value=KINP_FrntPTCRearRiActHeatPwr_W_ovrdval
  FrntPTCRiActHeatPwr : FVT_lib/inp/can_signal_template  SystemSampleTime=-1  VariantActivationTime=update diagram  Latency=0  AutoFrameSizeCalculation=off
      link override defval: Value=KINP_FrntPTCRiActHeatPwr_W_defval
      link override ovrdflg: Value=KINP_FrntPTCRiActHeatPwr_W_ovrdflg
      link override ovrdval: Value=KINP_FrntPTCRiActHeatPwr_W_ovrdval
  Terminator_{1..4} (4 alike) : Terminator
  True_VHAL_FrntPTCLeActHeatPwr_W : Constant  Value=TRUE  OutDataTypeStr=boolean
  True_VHAL_FrntPTCRearLeActHeatPwr_W : Constant  Value=TRUE  OutDataTypeStr=boolean
  True_VHAL_FrntPTCRearRiActHeatPwr_W : Constant  Value=TRUE  OutDataTypeStr=boolean
  True_VHAL_FrntPTCRiActHeatPwr_W : Constant  Value=TRUE  OutDataTypeStr=boolean
  slr1_{1..4} (4 alike) : BusSelector  OutputSignals=VINP_CANMsgValidzGWAPTC1_flg
  slr_VHAL_FrntPTCLeActHeatPwr_W : BusSelector  OutputSignals=VHAL_FrntPTCLeActHeatPwr_W
  slr_VHAL_FrntPTCRearLeActHeatPwr_W : BusSelector  OutputSignals=VHAL_FrntPTCRearLeActHeatPwr_W
  slr_VHAL_FrntPTCRearRiActHeatPwr_W : BusSelector  OutputSignals=VHAL_FrntPTCRearRiActHeatPwr_W
  slr_VHAL_FrntPTCRiActHeatPwr_W : BusSelector  OutputSignals=VHAL_FrntPTCRiActHeatPwr_W
  VINP_FrntPTCLeActHeatPwr_W : Outport
  VINP_FrntPTCRearLeActHeatPwr_W : Outport  Port=2
  VINP_FrntPTCRearRiActHeatPwr_W : Outport  Port=3
  VINP_FrntPTCRiActHeatPwr_W : Outport  Port=4
  wires:
  BHAL_outputs/1 -> [BHAL_outputs]
  inp_CanValid_bus/1 -> [inp_CanValid_bus]
  [BHAL_outputs] -> slr_VHAL_FrntPTCLeActHeatPwr_W/1
  slr_VHAL_FrntPTCLeActHeatPwr_W/1 -> FrntPTCLeActHeatPwr/1  "<VHAL_FrntPTCLeActHeatPwr_W>"
  True_VHAL_FrntPTCLeActHeatPwr_W/1 -> FrntPTCLeActHeatPwr/2
  [inp_CanValid_bus] -> slr1_1/1
  slr1_1/1 -> FrntPTCLeActHeatPwr/3  "<VINP_CANMsgValidzGWAPTC1_flg>"
  FrntPTCLeActHeatPwr/1 -> VINP_FrntPTCLeActHeatPwr_W/1  "VINP_FrntPTCLeActHeatPwr_W"
  FrntPTCLeActHeatPwr/2 -> Terminator_1/1
  [BHAL_outputs] -> slr_VHAL_FrntPTCRearLeActHeatPwr_W/1
  slr_VHAL_FrntPTCRearLeActHeatPwr_W/1 -> FrntPTCRearLeActHeatPwr/1  "<VHAL_FrntPTCRearLeActHeatPwr_W>"
  True_VHAL_FrntPTCRearLeActHeatPwr_W/1 -> FrntPTCRearLeActHeatPwr/2
  [inp_CanValid_bus] -> slr1_2/1
  slr1_2/1 -> FrntPTCRearLeActHeatPwr/3  "<VINP_CANMsgValidzGWAPTC1_flg>"
  FrntPTCRearLeActHeatPwr/1 -> VINP_FrntPTCRearLeActHeatPwr_W/1  "VINP_FrntPTCRearLeActHeatPwr_W"
  FrntPTCRearLeActHeatPwr/2 -> Terminator_2/1
  [BHAL_outputs] -> slr_VHAL_FrntPTCRearRiActHeatPwr_W/1
  slr_VHAL_FrntPTCRearRiActHeatPwr_W/1 -> FrntPTCRearRiActHeatPwr/1  "<VHAL_FrntPTCRearRiActHeatPwr_W>"
  True_VHAL_FrntPTCRearRiActHeatPwr_W/1 -> FrntPTCRearRiActHeatPwr/2
  [inp_CanValid_bus] -> slr1_3/1
  slr1_3/1 -> FrntPTCRearRiActHeatPwr/3  "<VINP_CANMsgValidzGWAPTC1_flg>"
  FrntPTCRearRiActHeatPwr/1 -> VINP_FrntPTCRearRiActHeatPwr_W/1  "VINP_FrntPTCRearRiActHeatPwr_W"
  FrntPTCRearRiActHeatPwr/2 -> Terminator_3/1
  [BHAL_outputs] -> slr_VHAL_FrntPTCRiActHeatPwr_W/1
  slr_VHAL_FrntPTCRiActHeatPwr_W/1 -> FrntPTCRiActHeatPwr/1  "<VHAL_FrntPTCRiActHeatPwr_W>"
  True_VHAL_FrntPTCRiActHeatPwr_W/1 -> FrntPTCRiActHeatPwr/2
  [inp_CanValid_bus] -> slr1_4/1
  slr1_4/1 -> FrntPTCRiActHeatPwr/3  "<VINP_CANMsgValidzGWAPTC1_flg>"
  FrntPTCRiActHeatPwr/1 -> VINP_FrntPTCRiActHeatPwr_W/1  "VINP_FrntPTCRiActHeatPwr_W"
  FrntPTCRiActHeatPwr/2 -> Terminator_4/1

== system inp/INP/CAN4/SignalCheck/zGW_CANFr1 ==
  BHAL_outputs : Inport
  inp_CanValid_bus : Inport  Port=2
  COMPActualPwr : FVT_lib/inp/can_signal_template  SystemSampleTime=-1  VariantActivationTime=update diagram  Latency=0  AutoFrameSizeCalculation=off
      link override defval: Value=KINP_COMPActualPwr_W_defval
      link override ovrdflg: Value=KINP_COMPActualPwr_W_ovrdflg
      link override ovrdval: Value=KINP_COMPActualPwr_W_ovrdval
  COMPConCur : FVT_lib/inp/can_signal_template  SystemSampleTime=-1  VariantActivationTime=update diagram  Latency=0  AutoFrameSizeCalculation=off
      link override defval: Value=KINP_COMPConCur_A_defval
      link override ovrdflg: Value=KINP_COMPConCur_A_ovrdflg
      link override ovrdval: Value=KINP_COMPConCur_A_ovrdval
  COMPConVolt : FVT_lib/inp/can_signal_template  SystemSampleTime=-1  VariantActivationTime=update diagram  Latency=0  AutoFrameSizeCalculation=off
      link override defval: Value=KINP_COMPConVolt_V_defval
      link override ovrdflg: Value=KINP_COMPConVolt_V_ovrdflg
      link override ovrdval: Value=KINP_COMPConVolt_V_ovrdval
  COMPStatorSpd : FVT_lib/inp/can_signal_template  SystemSampleTime=-1  VariantActivationTime=update diagram  Latency=0  AutoFrameSizeCalculation=off
      link override defval: Value=KINP_COMPStatorSpd_rpm_defval
      link override ovrdflg: Value=KINP_COMPStatorSpd_rpm_ovrdflg
      link override ovrdval: Value=KINP_COMPStatorSpd_rpm_ovrdval
  PTC1PowerConsumption : FVT_lib/inp/can_signal_template  SystemSampleTime=-1  VariantActivationTime=update diagram  Latency=0  AutoFrameSizeCalculation=off
      link override defval: Value=KINP_PTC1PowerConsumption_kW_defval
      link override ovrdflg: Value=KINP_PTC1PowerConsumption_kW_ovrdflg
      link override ovrdval: Value=KINP_PTC1PowerConsumption_kW_ovrdval
  Terminator_{1..5} (5 alike) : Terminator
  True_VHAL_COMPActualPwr_W : Constant  Value=TRUE  OutDataTypeStr=boolean
  True_VHAL_COMPConCur_A : Constant  Value=TRUE  OutDataTypeStr=boolean
  True_VHAL_COMPConVolt_V : Constant  Value=TRUE  OutDataTypeStr=boolean
  True_VHAL_COMPStatorSpd_rpm : Constant  Value=TRUE  OutDataTypeStr=boolean
  True_VHAL_PTC1PowerConsumption_kW : Constant  Value=TRUE  OutDataTypeStr=boolean
  slr1_{1..5} (5 alike) : BusSelector  OutputSignals=VINP_CANMsgValidzGWCANFr1_flg
  slr_VHAL_COMPActualPwr_W : BusSelector  OutputSignals=VHAL_COMPActualPwr_W
  slr_VHAL_COMPConCur_A : BusSelector  OutputSignals=VHAL_COMPConCur_A
  slr_VHAL_COMPConVolt_V : BusSelector  OutputSignals=VHAL_COMPConVolt_V
  slr_VHAL_COMPStatorSpd_rpm : BusSelector  OutputSignals=VHAL_COMPStatorSpd_rpm
  slr_VHAL_PTC1PowerConsumption_kW : BusSelector  OutputSignals=VHAL_PTC1PowerConsumption_kW
  VINP_COMPActualPwr_W : Outport
  VINP_COMPConCur_A : Outport  Port=2
  VINP_COMPConVolt_V : Outport  Port=3
  VINP_COMPStatorSpd_rpm : Outport  Port=4
  VINP_PTC1PowerConsumption_kW : Outport  Port=5
  wires:
  BHAL_outputs/1 -> [BHAL_outputs]
  inp_CanValid_bus/1 -> [inp_CanValid_bus]
  [BHAL_outputs] -> slr_VHAL_COMPActualPwr_W/1
  slr_VHAL_COMPActualPwr_W/1 -> COMPActualPwr/1  "<VHAL_COMPActualPwr_W>"
  True_VHAL_COMPActualPwr_W/1 -> COMPActualPwr/2
  [inp_CanValid_bus] -> slr1_1/1
  slr1_1/1 -> COMPActualPwr/3  "<VINP_CANMsgValidzGWCANFr1_flg>"
  COMPActualPwr/1 -> VINP_COMPActualPwr_W/1  "VINP_COMPActualPwr_W"
  COMPActualPwr/2 -> Terminator_1/1
  [BHAL_outputs] -> slr_VHAL_COMPConCur_A/1
  slr_VHAL_COMPConCur_A/1 -> COMPConCur/1  "<VHAL_COMPConCur_A>"
  True_VHAL_COMPConCur_A/1 -> COMPConCur/2
  [inp_CanValid_bus] -> slr1_2/1
  slr1_2/1 -> COMPConCur/3  "<VINP_CANMsgValidzGWCANFr1_flg>"
  COMPConCur/1 -> VINP_COMPConCur_A/1  "VINP_COMPConCur_A"
  COMPConCur/2 -> Terminator_2/1
  [BHAL_outputs] -> slr_VHAL_COMPConVolt_V/1
  slr_VHAL_COMPConVolt_V/1 -> COMPConVolt/1  "<VHAL_COMPConVolt_V>"
  True_VHAL_COMPConVolt_V/1 -> COMPConVolt/2
  [inp_CanValid_bus] -> slr1_3/1
  slr1_3/1 -> COMPConVolt/3  "<VINP_CANMsgValidzGWCANFr1_flg>"
  COMPConVolt/1 -> VINP_COMPConVolt_V/1  "VINP_COMPConVolt_V"
  COMPConVolt/2 -> Terminator_3/1
  [BHAL_outputs] -> slr_VHAL_COMPStatorSpd_rpm/1
  slr_VHAL_COMPStatorSpd_rpm/1 -> COMPStatorSpd/1  "<VHAL_COMPStatorSpd_rpm>"
  True_VHAL_COMPStatorSpd_rpm/1 -> COMPStatorSpd/2
  [inp_CanValid_bus] -> slr1_4/1
  slr1_4/1 -> COMPStatorSpd/3  "<VINP_CANMsgValidzGWCANFr1_flg>"
  COMPStatorSpd/1 -> VINP_COMPStatorSpd_rpm/1  "VINP_COMPStatorSpd_rpm"
  COMPStatorSpd/2 -> Terminator_4/1
  [BHAL_outputs] -> slr_VHAL_PTC1PowerConsumption_kW/1
  slr_VHAL_PTC1PowerConsumption_kW/1 -> PTC1PowerConsumption/1  "<VHAL_PTC1PowerConsumption_kW>"
  True_VHAL_PTC1PowerConsumption_kW/1 -> PTC1PowerConsumption/2
  [inp_CanValid_bus] -> slr1_5/1
  slr1_5/1 -> PTC1PowerConsumption/3  "<VINP_CANMsgValidzGWCANFr1_flg>"
  PTC1PowerConsumption/1 -> VINP_PTC1PowerConsumption_kW/1  "VINP_PTC1PowerConsumption_kW"
  PTC1PowerConsumption/2 -> Terminator_5/1
